simulink model "TelemetryInstruments"  (R2023b)
settings: Solver=VariableStepAuto  StartTime=0.0  StopTime=20  RelTol=1e-3
settings Model: PacingRate=0.500000  Creator=peter  LastModifiedBy=Pilot
settings ModelReferenceCC: EnableRefExpFcnMdlSchedulingChecks=on

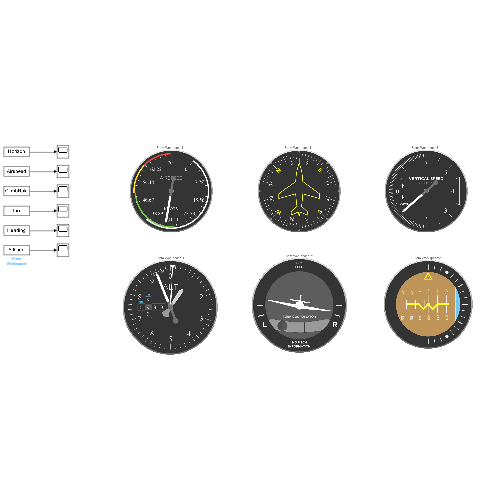
[thumbnail: Simulink's stored preview of the top-level diagram]
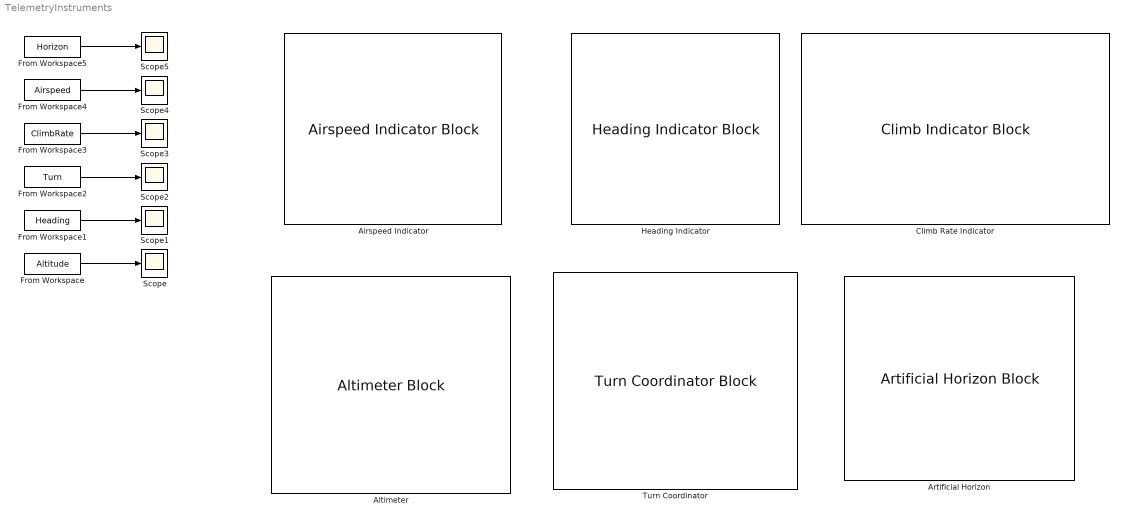
== system TelemetryInstruments ==
  Airspeed Indicator : AirspeedIndicatorBlock  ScaleMin=0  ScaleMax=70
  Altimeter : AltimeterBlock
  Artificial Horizon : ArtificialHorizonBlock
  Climb Rate Indicator : ClimbIndicatorBlock
  From Workspace : FromWorkspace  VariableName=Altitude
  From Workspace1 : FromWorkspace  VariableName=Heading
  From Workspace2 : FromWorkspace  VariableName=Turn
  From Workspace3 : FromWorkspace  VariableName=ClimbRate
  From Workspace4 : FromWorkspace  VariableName=Airspeed
  From Workspace5 : FromWorkspace  VariableName=Horizon
  Heading Indicator : HeadingIndicatorBlock
  Scope{,1..5} (6 alike) : Scope
  Turn Coordinator : TurnCoordinatorBlock
  wires:
  From Workspace/1 -> Scope/1
  From Workspace4/1 -> Scope4/1
  From Workspace3/1 -> Scope3/1
  From Workspace2/1 -> Scope2/1
  From Workspace1/1 -> Scope1/1
  From Workspace5/1 -> Scope5/1
